simulink model "CS637Assignment1_3"  (R2022a)
settings: Solver=VariableStepAuto  StartTime=0.0  StopTime=10.0  RelTol=1e-3
libraries: cstblocks x1
settings Model: Creator=kaush  LastModifiedBy=kaush

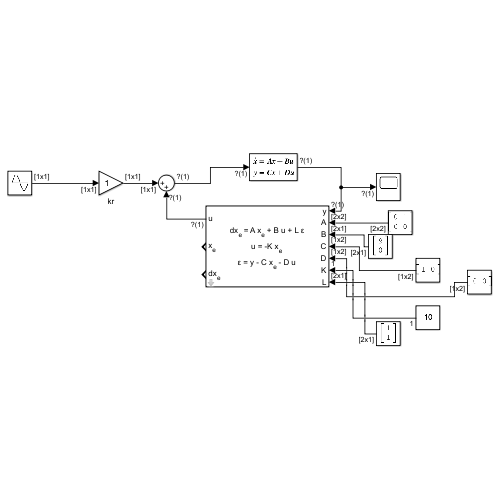
[thumbnail: Simulink's stored preview of the top-level diagram]
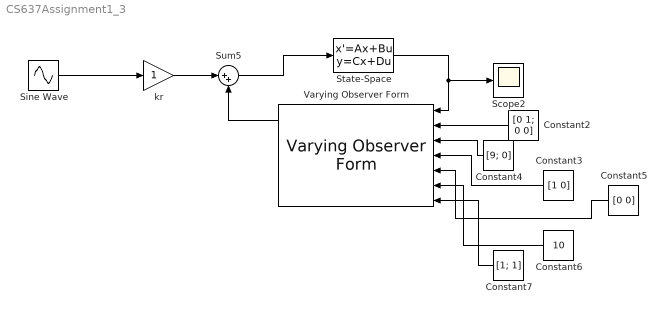
== system CS637Assignment1_3 ==
  Constant2 : Constant  Value=[0 1; 0 0]  VectorParams1D=off
  Constant3 : Constant  Value=[1 0]  VectorParams1D=off
  Constant4 : Constant  Value=[9; 0]  VectorParams1D=off
  Constant5 : Constant  Value=[0 0]  VectorParams1D=off
  Constant6 : Constant  Value=10
  Constant7 : Constant  Value=[1; 1]  VectorParams1D=off
  Scope2 : Scope
  Sine Wave : Sin  SampleTime=0  VectorParams1D=off
  State-Space : StateSpace  A=[0 1; 0 0]  B=[9; 0]  C=[1 0]  D=0  InitialCondition=0
  Sum5 : Sum  Inputs=|++
  Varying Observer Form : cstblocks/Linear Parameter Varying/Varying Observer Form  x0=0  xNames=''  OutputX=on  OutputDX=on
      settings: SourceProductBaseCode=CT
  kr : Gain
  wires:
  Constant4/1 -> Varying Observer Form/3
  Constant3/1 -> Varying Observer Form/4
  Constant5/1 -> Varying Observer Form/5
  Constant6/1 -> Varying Observer Form/6
  kr/1 -> Sum5/1
  State-Space/1 -> Varying Observer Form/1, Scope2/1
  Sine Wave/1 -> kr/1
  Varying Observer Form/1 -> Sum5/2
  Constant7/1 -> Varying Observer Form/7
  Constant2/1 -> Varying Observer Form/2
  Sum5/1 -> State-Space/1
